simulink model "deadbeat_smm_with_lqr"  (R2015a)
settings: Solver=FixedStepDiscrete  SolverMode=SingleTasking  StartTime=0.0  StopTime=inf  FixedStep=sample_time  RelTol=1e-3
undefined symbols (not defined in the file or in its folder): A_kalman_fourbar_gear, A_kalman_transverse, A_kalman_vertical, A_lpf_accelerometer, A_lpf_fourbar_angles, A_lpf_imu, A_lpf_lateral_angle, B1_lpf_accelerometer, B1_lpf_fourbar_angles, B1_lpf_imu, B1_lpf_lateral_angle, B2_lpf_accelerometer, B2_lpf_fourbar_angles, B2_lpf_imu, B2_lpf_lateral_angle, B_dx_versus_x0, B_kalman_fourbar_gear, B_kalman_transverse, B_kalman_vertical, backwards_K_sag_of_t, backwards_P_sag_of_t, C_kalman_fourbar_gear, C_kalman_transverse, C_kalman_vertical, com_leg_motor, com_torso, contact_threshold, control_start_time, d_ankle_to_foot, d_vertical_com, desired_com_forward_velocity, desired_com_lateral_velocity, desired_initial_leg_roll_left, desired_initial_leg_roll_right, desired_stance_beta2, desired_standing_torso_pitch, desired_standing_torso_roll, desired_standing_z, desired_torso_pitch, desired_torso_roll, Discrete, enable_bouncing, fcut_contact, fdesignblkfcn, forward_dx_of_dxstar, forward_x_of_dxstar, g, gcbh, HIP_MTR_MAX_CONT_TORQUE, HIP_MTR_MAX_TORQUE, i_leg_motor, i_robot, i_torso, initial_dx_estimate, initial_dy_estimate, initial_dz_estimate, initial_leg_selection, initial_z_estimate, k_lateral_accel_for_torso_roll, k_lateral_swing_on_boom ... (+77)
libraries: simulink x21, ctrlSharedLib x7, dsparch4 x3
(part 4 of 5)

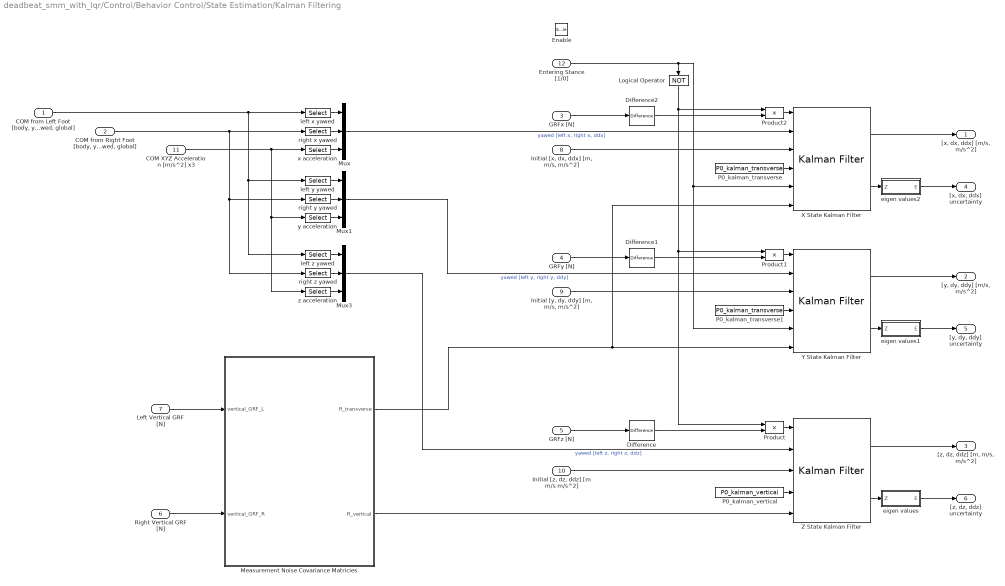
== system deadbeat_smm_with_lqr/Control/Behavior Control/State Estimation/Kalman Filtering ==
  "COM from Left Foot [body, yawed, global]" : Inport  SampleTime=sample_time
  "COM from Right Foot [body, yawed, global]" : Inport  Port=2  SampleTime=sample_time
  GRFx [N] : Inport  Port=3  SampleTime=sample_time
  GRFy [N] : Inport  Port=4  SampleTime=sample_time
  GRFz [N] : Inport  Port=5  SampleTime=sample_time
  Right Vertical GRF [N] : Inport  Port=6  SampleTime=sample_time
  Left Vertical GRF [N] : Inport  Port=7  SampleTime=sample_time
  "Initial [x, dx, ddx] [m, m/s, m/s^2]" : Inport  Port=8  PortDimensions=3  SampleTime=sample_time
  "Initial [y, dy, ddy] [m, m/s, m/s^2]" : Inport  Port=9  PortDimensions=3  SampleTime=sample_time
  "Initial [z, dz, ddz] [m m/s m/s^2]" : Inport  Port=10  PortDimensions=3  SampleTime=sample_time
  COM XYZ Acceleration [m/s^2] x3 : Inport  Port=11  SampleTime=sample_time
  Entering Stance [1/0] : Inport  Port=12  PortDimensions=1  SampleTime=sample_time
  Enable : EnablePort  StatesWhenEnabling=reset
  Difference : simulink/Discrete/Difference  ICPrevInput=0.0  InputProcessing=Inherited  OutMin=[]  OutMax=[]  OutDataType=fixdt(1, 16)  OutScaling=2^-10  DoSatur=off
  Difference1 : simulink/Discrete/Difference  ICPrevInput=0.0  InputProcessing=Inherited  OutMin=[]  OutMax=[]  OutDataType=fixdt(1, 16)  OutScaling=2^-10  DoSatur=off
  Difference2 : simulink/Discrete/Difference  ICPrevInput=0.0  InputProcessing=Inherited  OutMin=[]  OutMax=[]  OutDataType=fixdt(1, 16)  OutScaling=2^-10  DoSatur=off
  Logical Operator : Logic  Operator=NOT  AllPortsSameDT=off  OutDataTypeStr=boolean
  Measurement Noise Covariance Matricies : MATLAB Function  TreatAsAtomicUnit=on
  Mux : Mux  Inputs=3
  Mux1 : Mux  Inputs=3
  Mux3 : Mux  Inputs=3
  P0_kalman_transverse : Constant  Value=P0_kalman_transverse
  P0_kalman_transverse1 : Constant  Value=P0_kalman_transverse
  P0_kalman_vertical : Constant  Value=P0_kalman_vertical
  Product : Product
  Product1 : Product
  Product2 : Product
  X State Kalman Filter : ctrlSharedLib/Kalman Filter  TimeDomain=Discrete-Time  UseCurrentEstimator=on  ModelSource=Individual A, B, C, D matrices  ModelSourceVariable=A_kf  A=A_kalman_transverse  B=B_kalman_transverse  C=C_kalman_transverse  D=0  NumberOfStates=2  NumberOfInputs=1  NumberOfOutputs=2  InitialEstimateSource=Input port  X0=initial_dx_estimate  P0=P0_kalman_transverse  UseK=off  UseGH=on  NumberOfProcessNoiseInputs=1  G=G_kalman_transverse  TimeInvariantG=on  H=0  TimeInvariantH=on  Q=Q_kalman_GRF_difference  TimeInvariantQ=on  R=1  TimeInvariantR=off  N=0  TimeInvariantN=on  AddInputPort=on  AddEnablePort=off  ExternalReset=Rising  OutputEstimatedY=off  OutputP=on  Ts=sample_time
  Y State Kalman Filter : ctrlSharedLib/Kalman Filter  TimeDomain=Discrete-Time  UseCurrentEstimator=on  ModelSource=Individual A, B, C, D matrices  ModelSourceVariable=A_kf  A=A_kalman_transverse  B=B_kalman_transverse  C=C_kalman_transverse  D=0  NumberOfStates=2  NumberOfInputs=1  NumberOfOutputs=2  InitialEstimateSource=Input port  X0=initial_dy_estimate  P0=P0_kalman_transverse  UseK=off  UseGH=on  NumberOfProcessNoiseInputs=1  G=G_kalman_transverse  TimeInvariantG=on  H=0  TimeInvariantH=on  Q=Q_kalman_GRF_difference  TimeInvariantQ=on  R=1  TimeInvariantR=off  N=0  TimeInvariantN=on  AddInputPort=on  AddEnablePort=off  ExternalReset=Rising  OutputEstimatedY=off  OutputP=on  Ts=sample_time
  Z State Kalman Filter : ctrlSharedLib/Kalman Filter  TimeDomain=Discrete-Time  UseCurrentEstimator=on  ModelSource=Individual A, B, C, D matrices  ModelSourceVariable=A_kf  A=A_kalman_vertical  B=B_kalman_vertical  C=C_kalman_vertical  D=0  NumberOfStates=2  NumberOfInputs=1  NumberOfOutputs=2  InitialEstimateSource=Input port  X0=[initial_z_estimate; initial_dz_estimate]  P0=P0_kalman_vertical  UseK=off  UseGH=on  NumberOfProcessNoiseInputs=1  G=G_kalman_vertical  TimeInvariantG=on  H=0  TimeInvariantH=on  Q=Q_kalman_GRF_difference  TimeInvariantQ=on  R=1  TimeInvariantR=off  N=0  TimeInvariantN=on  AddInputPort=on  AddEnablePort=off  OutputEstimatedY=off  OutputP=on  Ts=sample_time
  eigen values : MATLAB Function  TreatAsAtomicUnit=on
  eigen values1 : MATLAB Function  TreatAsAtomicUnit=on
  eigen values2 : MATLAB Function  TreatAsAtomicUnit=on
  left x yawed : Selector  InputPortWidth=9  Indices=[4]
  left y yawed : Selector  InputPortWidth=9  Indices=[5]
  left z yawed : Selector  InputPortWidth=9  Indices=[6]
  right x yawed : Selector  InputPortWidth=9  Indices=[4]
  right y yawed : Selector  InputPortWidth=9  Indices=[5]
  right z yawed : Selector  InputPortWidth=9  Indices=[6]
  x acceleration : Selector  InputPortWidth=3  Indices=[1]
  y acceleration : Selector  InputPortWidth=3  Indices=[2]
  z acceleration : Selector  InputPortWidth=3  Indices=[3]
  "[x, dx, ddx] [m/s, m/s^2]" : Outport
  "[y, dy, ddy] [m/s, m/s^2]" : Outport  Port=2
  "[z, dz, ddz] [m, m/s, m/s^2]" : Outport  Port=3
  "[x, dx, ddx] uncertainty" : Outport  Port=4
  "[y, dy, ddy] uncertainty" : Outport  Port=5
  "[z, dz, ddz] uncertainty" : Outport  Port=6
  wires:
  X State Kalman Filter/1 -> "[x, dx, ddx] [m/s, m/s^2]"/1
  eigen values1/1(E) -> "[y, dy, ddy] uncertainty"/1
  eigen values2/1(E) -> "[x, dx, ddx] uncertainty"/1
  Y State Kalman Filter/1 -> "[y, dy, ddy] [m/s, m/s^2]"/1
  y acceleration/1 -> Mux1/3
  x acceleration/1 -> Mux/3
  z acceleration/1 -> Mux3/3
  COM XYZ Acceleration [m/s^2] x3/1 -> z acceleration/1, y acceleration/1, x acceleration/1
  Z State Kalman Filter/1 -> "[z, dz, ddz] [m, m/s, m/s^2]"/1
  GRFy [N]/1 -> Difference1/1
  Mux3/1 -> Z State Kalman Filter/2  "yawed [left z, right z, ddz]"
  GRFx [N]/1 -> Difference2/1
  Measurement Noise Covariance Matricies/2(R_vertical) -> Z State Kalman Filter/5
  Measurement Noise Covariance Matricies/1(R_transverse) -> X State Kalman Filter/6, Y State Kalman Filter/6
  Mux1/1 -> Y State Kalman Filter/2  "yawed [left y, right y, ddy]"
  Mux/1 -> X State Kalman Filter/2  "yawed [left x, right x, ddx]"
  Right Vertical GRF [N]/1 -> Measurement Noise Covariance Matricies/2(vertical_GRF_R)
  Left Vertical GRF [N]/1 -> Measurement Noise Covariance Matricies/1(vertical_GRF_L)
  "COM from Left Foot [body, yawed, global]"/1 -> left z yawed/1, left y yawed/1, left x yawed/1
  left x yawed/1 -> Mux/1
  "COM from Right Foot [body, yawed, global]"/1 -> right z yawed/1, right y yawed/1, right x yawed/1
  right x yawed/1 -> Mux/2
  left y yawed/1 -> Mux1/1
  right y yawed/1 -> Mux1/2
  left z yawed/1 -> Mux3/1
  right z yawed/1 -> Mux3/2
  P0_kalman_transverse/1 -> X State Kalman Filter/4
  "Initial [x, dx, ddx] [m, m/s, m/s^2]"/1 -> X State Kalman Filter/3
  P0_kalman_transverse1/1 -> Y State Kalman Filter/4
  "Initial [y, dy, ddy] [m, m/s, m/s^2]"/1 -> Y State Kalman Filter/3
  P0_kalman_vertical/1 -> Z State Kalman Filter/4
  "Initial [z, dz, ddz] [m m/s m/s^2]"/1 -> Z State Kalman Filter/3
  X State Kalman Filter/2 -> eigen values2/1(Z)
  Y State Kalman Filter/2 -> eigen values1/1(Z)
  Z State Kalman Filter/2 -> eigen values/1(Z)
  eigen values/1(E) -> "[z, dz, ddz] uncertainty"/1
  Logical Operator/1 -> Product2/1, Product/1, Product1/1
  Difference/1 -> Product/2
  Entering Stance [1/0]/1 -> Y State Kalman Filter/5, X State Kalman Filter/5, Logical Operator/1
  Difference1/1 -> Product1/2
  Difference2/1 -> Product2/2
  Product2/1 -> X State Kalman Filter/1
  Product1/1 -> Y State Kalman Filter/1
  Product/1 -> Z State Kalman Filter/1
  GRFz [N]/1 -> Difference/1

== system deadbeat_smm_with_lqr/Control/Behavior Control/State Estimation/Lowpass Filter ==
  In : Inport
  Generated Filter Block : dsparch4/Biquad Filter  Tag=BlockMethodSubSystem  IIRFiltStruct=Direct form II  CoeffSource=Specify via dialog  BiQuadCoeffs=[1.0218648663828083 -2 1.0218648663828083 1 -1.9114378222117407 0.91557643487411833]  a0Flag=Warning  IC=0  ICnum=0  ICden=0  denAccumFracLength=30  denProdOutputFracLength=30  secondMemoryFracLength=15  roundingMode=Floor  overflowMode=off  ScaleValues=[0.0041174265739107223;22.985401576126357]  optimizeScaleValues=off  ScaleValueMode=Specify via input port (g)  scaleValueFracLength=14  FilterSource=Specify via dialog  FilterObject=Hm_biquad
  Out : Outport
  wires:
  In/1 -> Generated Filter Block/1
  Generated Filter Block/1 -> Out/1

== system deadbeat_smm_with_lqr/Control/Behavior Control/Primary and Lateral Behavior/Circular Buffer/Enabled on Touchdown ==
  In : Inport
  Enable : EnablePort
  Out : Outport
  wires:
  In/1 -> Out/1

== system deadbeat_smm_with_lqr/Control/Behavior Control/Primary and Lateral Behavior/Flight/Back//Front PD ==
  Desired Position [rad] [back front] : Inport
  Desired Velocity [rad/s] [back front] : Inport  Port=2
  Measured Position [rad] [back front] : Inport  Port=3
  Measured Velocity [rad/s] [back front] : Inport  Port=4
  Back Tracking : Scope  NumInputPorts=2
      settings: YMin=3.725~-1  YMax=4.05~0.9  SaveName=ScopeData6  SampleInput=on
  Front Tracking : Scope  NumInputPorts=2
      settings: YMin=-1~-0.8  YMax=1~1.4  SaveName=ScopeData31  SampleInput=on
  Kp_SEA_Trajectory : Constant  Value=kp_velocity_swing_trajectory
  Mux{1..2,12..13} (4 alike) : Mux  Inputs=2
  Product1 : Product
  Selector{,1..3} (4 alike) : Selector  InputPortWidth=2  Indices=[1]
  Selector{4..7} (4 alike) : Selector  InputPortWidth=2  Indices=[2]
  Sum7 : Sum  Inputs=|+-
  Sum9 : Sum
  Commanded Velocity [rad/s] [back front] : Outport
  wires:
  Kp_SEA_Trajectory/1 -> Product1/2
  Sum9/1 -> Commanded Velocity [rad/s] [back front]/1
  Measured Velocity [rad/s] [back front]/1 -> Selector7/1, Selector3/1
  Desired Velocity [rad/s] [back front]/1 -> Selector6/1, Selector2/1, Sum9/2
  Measured Position [rad] [back front]/1 -> Selector4/1, Selector/1, Sum7/2
  Sum7/1 -> Product1/1
  Product1/1 -> Sum9/1
  Mux12/1 -> Back Tracking/2
  Mux13/1 -> Back Tracking/1
  Desired Position [rad] [back front]/1 -> Selector5/1, Selector1/1, Sum7/1
  Mux1/1 -> Front Tracking/2
  Mux2/1 -> Front Tracking/1
  Selector/1 -> Mux13/1
  Selector1/1 -> Mux13/2
  Selector2/1 -> Mux12/1
  Selector3/1 -> Mux12/2
  Selector5/1 -> Mux2/2
  Selector4/1 -> Mux2/1
  Selector6/1 -> Mux1/1
  Selector7/1 -> Mux1/2

== system deadbeat_smm_with_lqr/Control/Behavior Control/Primary and Lateral Behavior/Flight/Hold Values on Takeoff ==
  in : Inport
  Trigger : TriggerPort  ShowOutputPort=on  PortDimensions=1
  Subsystem : Subsystem
  out : Outport
  wires:
  in/1 -> Subsystem/1(in)
  Subsystem/1(out) -> out/1
  Trigger/1 -> Subsystem/Enable

== system deadbeat_smm_with_lqr/Control/Behavior Control/Primary and Lateral Behavior/Stance/Chirp Frequency ==
  Time Since Stance : Inport
  Chirp Freq Factor Saturation : Saturate  UpperLimit=standing_bounce_max_chirp_scale  LowerLimit=0
      settings: AttributesFormatString=Top: %<UpperLimit>\nBottom: %<LowerLimit>
  Compare To Constant1 : simulink/Logic and Bit Operations/Compare To Constant  relop=~=  const=standing_bounce_max_chirp_scale  OutDataTypeStr=boolean
  Constant1 : Constant
  Constant5 : Constant  Value=standing_bounce_increase_rate
  Product{1..4} (4 alike) : Product
  Sum : Sum  Inputs=++|
  standing_bounce_frequency : Constant  Value=standing_bounce_frequency
  w : Outport
  dw/dt : Outport  Port=2
  wires:
  standing_bounce_frequency/1 -> Product2/1, Product3/1
  Chirp Freq Factor Saturation/1 -> Product3/2, Compare To Constant1/1
  Product3/1 -> w/1
  Product1/1 -> dw/dt/1
  Compare To Constant1/1 -> Product1/1
  Product2/1 -> Product1/2
  Constant5/1 -> Product2/2, Product4/2
  Time Since Stance/1 -> Product4/1
  Sum/1 -> Chirp Freq Factor Saturation/1
  Product4/1 -> Sum/2
  Constant1/1 -> Sum/1

== system deadbeat_smm_with_lqr/Control/Behavior Control/Primary and Lateral Behavior/Stance/Compute Forces1 ==
  XYZ Acceleration : Inport
  Constant5 : Constant  Value=g
  Demux : Demux  Outputs=3
  Gain4 : Gain  Gain=m_total_real
  Mux : Mux  Inputs=3
  Sum8 : Sum  Inputs=|++
  XYZ Force : Outport
  wires:
  Constant5/1 -> Sum8/2
  XYZ Acceleration/1 -> Demux/1
  Gain4/1 -> XYZ Force/1
  Mux/1 -> Gain4/1
  Sum8/1 -> Mux/3
  Demux/3 -> Sum8/1
  Demux/2 -> Mux/2
  Demux/1 -> Mux/1

== system deadbeat_smm_with_lqr/Control/Behavior Control/Primary and Lateral Behavior/Stance/Hold Values on Takeoff ==
  in : Inport
  Trigger : TriggerPort  ShowOutputPort=on  PortDimensions=1
  Subsystem : Subsystem
  out : Outport
  wires:
  Trigger/1 -> Subsystem/Enable
  Subsystem/1(out) -> out/1
  in/1 -> Subsystem/1(in)

== system deadbeat_smm_with_lqr/Control/Behavior Control/Primary and Lateral Behavior/Stance/Hold Values on Touchdown ==
  in : Inport
  Trigger : TriggerPort  ShowOutputPort=on  PortDimensions=1
  Subsystem : Subsystem
  out : Outport
  wires:
  in/1 -> Subsystem/1(in)
  Subsystem/1(out) -> out/1
  Trigger/1 -> Subsystem/Enable

== system deadbeat_smm_with_lqr/Control/Behavior Control/Primary and Lateral Behavior/Stance/Lowpass Filter ==
  In : Inport
  Generated Filter Block : dsparch4/Biquad Filter  Tag=BlockMethodSubSystem  IIRFiltStruct=Direct form II  CoeffSource=Specify via dialog  BiQuadCoeffs=[1.2169083457291219 -2 1.2169083457291219 1 -1.7334293610249598 0.76768521888208641]  a0Flag=Warning  IC=0  ICnum=0  ICden=0  denAccumFracLength=30  denProdOutputFracLength=30  secondMemoryFracLength=15  roundingMode=Floor  overflowMode=off  ScaleValues=[0.034049223021428709;2.3191101889079508]  optimizeScaleValues=off  ScaleValueMode=Specify via input port (g)  scaleValueFracLength=14  FilterSource=Specify via dialog  FilterObject=Hm_biquad
  Out : Outport
  wires:
  In/1 -> Generated Filter Block/1
  Generated Filter Block/1 -> Out/1

== system deadbeat_smm_with_lqr/Control/Behavior Control/Primary and Lateral Behavior/Stance/Torque Distribution ==
  Leg Torque [Nm] : Inport
  Leg Force [N] : Inport  Port=2
  w [m] : Inport  Port=3
  Gain : Gain  Gain=0.5
  Gain1 : Gain  Gain=0.5
  Motor Torque Saturation Optimization : MATLAB Function  TreatAsAtomicUnit=on
  Product : Product  RndMeth=Zero
  Sum : Sum  Inputs=|++
  Sum1 : Sum  Inputs=+-|
  Back Torque [Nm] : Outport
  Front Torque [Nm] : Outport  Port=2
  wires:
  Gain/1 -> Motor Torque Saturation Optimization/1(x1s)
  Gain1/1 -> Motor Torque Saturation Optimization/2(x2s)
  Product/1 -> Gain1/1
  Leg Force [N]/1 -> Product/1
  Motor Torque Saturation Optimization/2(t2) -> Sum/2, Sum1/2
  w [m]/1 -> Product/2
  Motor Torque Saturation Optimization/1(t1) -> Sum1/1, Sum/1
  Sum/1 -> Front Torque [Nm]/1
  Leg Torque [Nm]/1 -> Gain/1
  Sum1/1 -> Back Torque [Nm]/1

== system deadbeat_smm_with_lqr/Control/Behavior Control/Primary and Lateral Behavior/Flight/Hold Values on Takeoff/Subsystem ==
  in : Inport
  Enable : EnablePort
  out : Outport
  wires:
  in/1 -> out/1

== system deadbeat_smm_with_lqr/Control/Behavior Control/Primary and Lateral Behavior/Stance/Hold Values on Takeoff/Subsystem ==
  in : Inport
  Enable : EnablePort
  out : Outport
  wires:
  in/1 -> out/1

== system deadbeat_smm_with_lqr/Control/Behavior Control/Primary and Lateral Behavior/Stance/Hold Values on Touchdown/Subsystem ==
  in : Inport
  Enable : EnablePort
  out : Outport
  wires:
  in/1 -> out/1

== matlab function deadbeat_smm_with_lqr/Control/Behavior Control/Compute World Frame COM Coordinates from Yawed Frame ==
  data: com_position_world output; X_dX input; Y_dY input; Z_dZ input; torso_yaw input; com_velocity_world output
function [com_position_world, com_velocity_world] ...
          = compute_com_state_in_world_frame(X_dX, Y_dY, Z_dZ, torso_yaw)

    R_yawed_to_world = R_yaw(torso_yaw(1));
    dR_yawed_to_world = dR_yaw(torso_yaw(1),torso_yaw(2));
    
    com_position_yawed = [X_dX(1); Y_dY(1); Z_dZ(1)];
    com_velocity_yawed = [X_dX(2); Y_dY(2); Z_dZ(2)];
    
    com_position_world = R_yawed_to_world*com_position_yawed;
    com_velocity_world = dR_yawed_to_world*com_position_yawed + R_yawed_to_world*com_velocity_yawed;

end

function R_gy = R_yaw(psi) % map yawed frame to global
  R_gy = [cos(psi), -sin(psi), 0; sin(psi), cos(psi), 0; 0 0 1]; 
end
function dR_gy = dR_yaw(psi,dpsi)
  dR_gy = dpsi*[-sin(psi), -cos(psi), 0; cos(psi), -sin(psi), 0; 0 0 0];
end

== matlab function deadbeat_smm_with_lqr/Control/Behavior Control/Primary and Lateral Behavior/Stance/2D Lateral Stance Control ==
  data: F_leg input; lateral_torque output; lateral_offset parameter; m_total_real parameter; m_leg_motor parameter; m_leg parameter
function lateral_torque = lateralStanceControl2D(F_leg,lateral_offset,m_total_real,m_leg_motor,m_leg)
    lateral_torque = -F_leg*lateral_offset*(m_total_real-(m_leg_motor+m_leg))/m_total_real;
end

== matlab function deadbeat_smm_with_lqr/Control/Behavior Control/Atrias Swing control/Avoid Hitting Mechanical Limits ==
  data: back_cmd output double; front_cmd output double; dback_cmd output double; dfront_cmd output double; ddback_cmd output double; ddfront_cmd output double; back_desired input; dback_desired input; ddback_desired input; front_desired input; dfront_desired input; ddfront_desired input; min_front_bar_angle parameter; max_front_bar_angle parameter; min_back_bar_angle parameter; max_back_bar_angle parameter
%% Avoid joint limits by ensuring we don't command velocities/accelerations that would push us into them when we are close to them.
function [back_cmd, front_cmd, dback_cmd, dfront_cmd, ddback_cmd, ddfront_cmd] ...
    = AvoidFourbarLimits(back_desired,dback_desired, ddback_desired, ...
          front_desired, dfront_desired, ddfront_desired, ...
          min_front_bar_angle, max_front_bar_angle, min_back_bar_angle, max_back_bar_angle)
    [back_cmd, front_cmd, dback_cmd, dfront_cmd, ddback_cmd, ddfront_cmd] = AvoidFourbarLimits(back_desired,dback_desired, ddback_desired, front_desired, dfront_desired, ddfront_desired, min_front_bar_angle, max_front_bar_angle, min_back_bar_angle, max_back_bar_angle);
end

== matlab function deadbeat_smm_with_lqr/Control/Behavior Control/Atrias Swing control/Convert COM Position to Joint Angles + Leg Length  ==
  data: desired_leg_length output; X_star input; Y_star input; Z_star input; right_left input; com_pelvis_body input; desired_alpha output; desired_beta output; dcom_pelvis_body input; roll input; pitch input; sagittal_angle input; lateral_angle input; leg_length input; lateral_offset parameter; minimum_lateral_beta parameter; maximum_lateral_beta parameter
function [ desired_leg_length, desired_alpha, desired_beta ]  =  ...
          ConvertToJointAnglesAndLegLength(X_star, Y_star, Z_star, right_left,...
                           com_pelvis_body, dcom_pelvis_body, ...
                           roll, pitch, sagittal_angle, lateral_angle, leg_length,...
                           lateral_offset, minimum_lateral_beta, maximum_lateral_beta) 

    q = [roll(1), pitch(1), sagittal_angle(1), lateral_angle(1), leg_length(1)];
    dq = [roll(2), pitch(2), sagittal_angle(2), lateral_angle(2), leg_length(2)];
    [desired_alpha, desired_beta, desired_leg_length]  =  ConvertComPositionToLegAnglesAndLegLength(X_star, Y_star, Z_star, right_left, com_pelvis_body, dcom_pelvis_body, q, dq, lateral_offset);   
    desired_beta = saturate(desired_beta, minimum_lateral_beta, maximum_lateral_beta);
end

function [desired_saturated] = saturate(desired, minimum_lateral_beta, maximum_lateral_beta)
    desired_saturated = desired;
    if desired(1) < minimum_lateral_beta
        desired_saturated = [minimum_lateral_beta; 0; 0];
    elseif desired(1) > maximum_lateral_beta
        desired_saturated = [maximum_lateral_beta; 0; 0];    
    end
end

== matlab function deadbeat_smm_with_lqr/Control/Behavior Control/Atrias Swing control/Virtual Leg to Four Bar ==
  data: l_leg input; dl_leg input; ddl_leg input; phi input; dphi input; ddphi input; back output; dback output; ddback output; front output; dfront output; ddfront output
function [back, dback, ddback, front, dfront, ddfront] = VirtualLegToFourBar(l_leg, dl_leg, ddl_leg, phi, dphi, ddphi)
    [back, dback, ddback, front, dfront, ddfront] = VirtualLegToFourBar(l_leg, dl_leg, ddl_leg, phi, dphi, ddphi);
end

== stateflow chart deadbeat_smm_with_lqr/Control/Behavior Control/Contact State Machine/State Machine ==
  state TouchDown
  state LockedContact
  state Unloading
  state Takeoff
  state Flight
  (junction 91) -> TouchDown
  TouchDown -> (junction 130) [order 2] : [vertical_grf < contact_threshold]
  (junction 93) -> (junction 91)
  (junction 130) -> (junction 128)
  TouchDown -> LockedContact [order 1] : [vertical_grf > loaded_threshold]
  (junction 115) -> LockedContact
  (junction 118) -> (junction 115)
  LockedContact -> Unloading : [z_velocity >= 0 && previous_z_velocity < 0]
  Unloading -> LockedContact [order 2] : [vertical_grf > loaded_threshold && z_velocity < 0]
  (junction 122) -> (junction 118)
  Unloading -> Takeoff [order 1] : [vertical_grf < contact_threshold]
  Takeoff -> Flight : after(t_flight,sec)
  (default) -> Flight
  Flight -> (junction 93) : [vertical_grf > contact_threshold]
  (junction 128) -> Flight
  data: z_velocity input; previous_z_velocity input; vertical_grf input; t_flight parameter; g parameter; contact_threshold parameter; loaded_threshold parameter; TouchDown output boolean; LockedContact output boolean; Unloading output boolean; Takeoff output boolean; Flight output boolean; vertical_acceleration input

== matlab function deadbeat_smm_with_lqr/Control/Behavior Control/Force Estimation/3D Forward Dynamics yawed ==
  data: right_or_left input; torso_roll input size=2; torso_pitch input double size=2; torso_yaw input double size=2; primary_sagittal_leg_angle input double size=2; primary_leg_length input double size=2; primary_leg_roll input double size=2; secondary_leg_roll input double size=2; primary_leg_torque input; primary_leg_force input; primary_lateral_torque input; secondary_lateral_torque input; R_GRF output double size=3; L_GRF output size=3; ddroll output double; g parameter; m_leg_motor parameter; m_torso parameter; i_torso parameter; i_leg_motor parameter; lateral_offset parameter; com_torso parameter; torso_centerline_roll_offset_angle parameter
%% Forward 3D ATRIAS dynamics
function [R_GRF, L_GRF, ddroll]  =  ForwardDynamics3D(right_or_left, ...
                                                      torso_roll, torso_pitch, torso_yaw, ...
                                                      primary_sagittal_leg_angle, primary_leg_length,...
                                                      primary_leg_roll, secondary_leg_roll, ...
                                                      primary_leg_torque, primary_leg_force, ...
                                                      primary_lateral_torque, secondary_lateral_torque, ...
                                                      g, m_leg_motor, m_torso, i_torso, i_leg_motor, lateral_offset, com_torso, torso_centerline_roll_offset_angle)

    d = norm(com_torso(2:3));
    It = mean(i_torso);
    Im = mean(i_leg_motor);
    
    phi    = torso_roll(1) + torso_centerline_roll_offset_angle;  % roll
    theta  = torso_pitch(1);                   % pitch
    alpha1 = primary_sagittal_leg_angle(1);    % primary sagittal leg angle
    beta1  = primary_leg_roll(1);              % primary leg roll
    beta2  = secondary_leg_roll(1);            % secondary leg roll
    if right_or_left
        beta1 = beta1 - torso_centerline_roll_offset_angle;
        beta2 = beta2 + torso_centerline_roll_offset_angle;
    else
        beta1 = beta1 + torso_centerline_roll_offset_angle;
        beta2 = beta2 - torso_centerline_roll_offset_angle;
    end 
    l1     = primary_leg_length(1);            % primary leg length
    
    dphi    = torso_roll(2);
    dtheta  = torso_pitch(2);
    dpsi    = torso_yaw(2);
    dalpha1 = primary_sagittal_leg_angle(2);
    dbeta1  = primary_leg_roll(2);
    dbeta2  = secondary_leg_roll(2);
    dl1     = primary_leg_length(2);
    
    
    tau_a1 = primary_leg_torque;
    tau_b1 = primary_lateral_torque;
    tau_b2 = secondary_lateral_torque;
    F_l1 = primary_leg_force;

    if right_or_left == 1
      A = A_fwd_yawed_right(lateral_offset,d,m_leg_motor,m_torso,It,Im,phi,theta,alpha1,beta1,beta2,l1);
      B = B_fwd_yawed_right(lateral_offset,d,g,m_leg_motor,m_torso,It,Im,phi,theta,alpha1,beta1,beta2,l1,dphi,dtheta,dpsi,dalpha1,dbeta1,dbeta2,dl1,tau_a1,tau_b1,tau_b2,F_l1);
    else
      A = A_fwd_yawed_left(lateral_offset,d,m_leg_motor,m_torso,It,Im,phi,theta,alpha1,beta1,beta2,l1);
      B = B_fwd_yawed_left(lateral_offset,d,g,m_leg_motor,m_torso,It,Im,phi,theta,alpha1,beta1,beta2,l1,dphi,dtheta,dpsi,dalpha1,dbeta1,dbeta2,dl1,tau_a1,tau_b1,tau_b2,F_l1);
    end
    
    x_fwd = A \ B;
    ddroll = x_fwd(4);
    GRF = zeros(3,1);
    GRF(1) = x_fwd(11);
    GRF(2) = x_fwd(12);
    GRF(3) = x_fwd(13); 
    
    if right_or_left == 1
        R_GRF = GRF;
        L_GRF = [0;0;0];
    else
        R_GRF = [0;0;0];
        L_GRF = GRF;
    end
end

== matlab function deadbeat_smm_with_lqr/Control/Behavior Control/Force Estimation/Leg Force Measurements/Nonlinear Spring Force ==
  data: deflections input; tau_sea output
function tau_sea   = SeaSpringForce( deflections )
    tau_sea = SeaSpringForce( deflections );
end

== matlab function deadbeat_smm_with_lqr/Control/Behavior Control/Knee Torques ==
  data: right_knees_to_foot input; right_front_knee_torques_from_fd output; left_knees_to_foot input; grf_from_seas input; grf_from_accelerometer input; right_back_knee_torques_from_fd output; right_front_knee_torques_from_accelerometer output; right_back_knee_torques_from_accelerometer output; left_front_knee_torques_from_fd output; left_back_knee_torques_from_fd output; left_front_knee_torques_from_accelerometer output; left_back_knee_torques_from_accelerometer output
function [right_front_knee_torques_from_fd, right_back_knee_torques_from_fd,...
          right_front_knee_torques_from_accelerometer, right_back_knee_torques_from_accelerometer,...
          left_front_knee_torques_from_fd, left_back_knee_torques_from_fd,...
          left_front_knee_torques_from_accelerometer, left_back_knee_torques_from_accelerometer] ...
          = compute_knee_torques(right_knees_to_foot, left_knees_to_foot, grf_from_seas, grf_from_accelerometer)

      right_front_knee_torques_from_fd = cross(right_knees_to_foot(1:3), grf_from_seas);
      right_back_knee_torques_from_fd = cross(right_knees_to_foot(4:6), grf_from_seas);
      right_front_knee_torques_from_accelerometer = cross(right_knees_to_foot(1:3), grf_from_accelerometer);
      right_back_knee_torques_from_accelerometer = cross(right_knees_to_foot(4:6), grf_from_accelerometer);
      
      left_front_knee_torques_from_fd = cross(left_knees_to_foot(1:3), grf_from_seas);
      left_back_knee_torques_from_fd = cross(left_knees_to_foot(4:6), grf_from_seas);
      left_front_knee_torques_from_accelerometer = cross(left_knees_to_foot(1:3), grf_from_accelerometer);
      left_back_knee_torques_from_accelerometer = cross(left_knees_to_foot(4:6), grf_from_accelerometer);
end

== matlab function deadbeat_smm_with_lqr/Control/Behavior Control/Primary Secondary Leg Swap/ToggleRightLeftLeg ==
  data: toggle input boolean; right_left output double; previous_right_left input double
function right_left = ToggleRightLeftLeg(toggle, previous_right_left)
    
    if toggle
        right_left = -previous_right_left + 1;
    else
        right_left = previous_right_left;
    end

end

== matlab function deadbeat_smm_with_lqr/Control/Behavior Control/Primary and Lateral Behavior/Circular Buffer/Buffer ==
  data: data input; buffer output size=recorded_steps; trigger input; buffer_size input
function buffer  = buffer_data(data, trigger, buffer_size)

    persistent buffer_memory
    coder.varsize('buffer_memory',100);
    if isempty(buffer_memory)
        buffer_memory = [];
    end
    
    if trigger
        buffer_memory = [data; buffer_memory];
        if size(buffer_memory, 1) > buffer_size
            buffer_memory = buffer_memory(1:buffer_size,:);
        end
    end
    
    buffer = buffer_memory;

end

== matlab function deadbeat_smm_with_lqr/Control/Behavior Control/Primary and Lateral Behavior/Circular Buffer/Buffer1 ==
  data: data input; buffer output size=recorded_steps; trigger input; buffer_size input
function buffer  = buffer_data(data, trigger, buffer_size)

    persistent buffer_memory
    coder.varsize('buffer_memory',100);
    if isempty(buffer_memory)
        buffer_memory = [];
    end
    
    if trigger
        buffer_memory = [data; buffer_memory];
        if size(buffer_memory, 1) > buffer_size
            buffer_memory = buffer_memory(1:buffer_size,:);
        end
    end
    
    buffer = buffer_memory;

end

== matlab function deadbeat_smm_with_lqr/Control/Behavior Control/Primary and Lateral Behavior/Circular Buffer/Buffer2 ==
  data: data input; buffer output size=recorded_steps; trigger input; buffer_size input
function buffer  = buffer_data(data, trigger, buffer_size)

    persistent buffer_memory
    coder.varsize('buffer_memory',100);
    if isempty(buffer_memory)
        buffer_memory = [];
    end
    
    if trigger
        buffer_memory = [data; buffer_memory];
        if size(buffer_memory, 1) > buffer_size
            buffer_memory = buffer_memory(1:buffer_size,:);
        end
    end
    
    buffer = buffer_memory;

end

== matlab function deadbeat_smm_with_lqr/Control/Behavior Control/Primary and Lateral Behavior/Circular Buffer/Buffer3 ==
  data: data input; buffer output size=recorded_steps; trigger input; buffer_size input
function buffer  = buffer_data(data, trigger, buffer_size)

    persistent buffer_memory
    coder.varsize('buffer_memory',100);
    if isempty(buffer_memory)
        buffer_memory = [];
    end
    
    if trigger
        buffer_memory = [data; buffer_memory];
        if size(buffer_memory, 1) > buffer_size
            buffer_memory = buffer_memory(1:buffer_size,:);
        end
    end
    
    buffer = buffer_memory;

end

== matlab function deadbeat_smm_with_lqr/Control/Behavior Control/Primary and Lateral Behavior/Circular Buffer/Buffer4 ==
  data: data input; buffer output size=recorded_steps; trigger input; buffer_size input
function buffer  = buffer_data(data, trigger, buffer_size)

    persistent buffer_memory
    coder.varsize('buffer_memory',100);
    if isempty(buffer_memory)
        buffer_memory = [];
    end
    
    if trigger
        buffer_memory = [data; buffer_memory];
        if size(buffer_memory, 1) > buffer_size
            buffer_memory = buffer_memory(1:buffer_size,:);
        end
    end
    
    buffer = buffer_memory;

end

== matlab function deadbeat_smm_with_lqr/Control/Behavior Control/Primary and Lateral Behavior/Circular Buffer/Buffer5 ==
  data: data input; buffer output size=recorded_steps; trigger input; buffer_size input
function buffer  = buffer_data(data, trigger, buffer_size)

    persistent buffer_memory
    coder.varsize('buffer_memory',100);
    if isempty(buffer_memory)
        buffer_memory = [];
    end
    
    if trigger
        buffer_memory = [data; buffer_memory];
        if size(buffer_memory, 1) > buffer_size
            buffer_memory = buffer_memory(1:buffer_size,:);
        end
    end
    
    buffer = buffer_memory;

end

== matlab function deadbeat_smm_with_lqr/Control/Behavior Control/Primary and Lateral Behavior/Circular Buffer/Buffer6 ==
  data: data input; buffer output size=recorded_steps; trigger input; buffer_size input
function buffer  = buffer_data(data, trigger, buffer_size)

    persistent buffer_memory
    coder.varsize('buffer_memory',100);
    if isempty(buffer_memory)
        buffer_memory = [];
    end
    
    if trigger
        buffer_memory = [data; buffer_memory];
        if size(buffer_memory, 1) > buffer_size
            buffer_memory = buffer_memory(1:buffer_size,:);
        end
    end
    
    buffer = buffer_memory;

end

== matlab function deadbeat_smm_with_lqr/Control/Behavior Control/Primary and Lateral Behavior/Circular Buffer/Buffer7 ==
  data: data input; buffer output size=recorded_steps; trigger input; buffer_size input
function buffer  = buffer_data(data, trigger, buffer_size)

    persistent buffer_memory
    coder.varsize('buffer_memory',100);
    if isempty(buffer_memory)
        buffer_memory = [];
    end
    
    if trigger
        buffer_memory = [data; buffer_memory];
        if size(buffer_memory, 1) > buffer_size
            buffer_memory = buffer_memory(1:buffer_size,:);
        end
    end
    
    buffer = buffer_memory;

end

== matlab function deadbeat_smm_with_lqr/Control/Behavior Control/Primary and Lateral Behavior/Closed Loop Compensation/CLOSED LOOP COMPENSATION X FOR VAIRABLE SPEED ==
  data: A_cl input; epsilon input; c input; delta_s_i input; dx_star input; B_cl input; delta_ux output
function delta_ux  = closed_loop_compensation_dxstar...
         (A_cl,epsilon, c, delta_s_i, dx_star, B_cl)
% assume form of delta_s_{i+1} = A_cl*delta_s_i + epsilon +c*dx_star + B_cl*delta_ux
% where delta measures deviation from deadbeat case. solve for
% delta_ux = (-A_cl*delta_s_i-epsilon - c*dxstar)/B_cl to achieve deadbeat
delta_ux = (-A_cl*delta_s_i - epsilon - c*dx_star)/B_cl;

== matlab function deadbeat_smm_with_lqr/Control/Behavior Control/Primary and Lateral Behavior/Closed Loop Compensation/CLOSED LOOP COMPENSATION Y FOR VAIRABLE SPEED ==
  data: A_cl input; epsilon input; c input; delta_s_i input; dx_star input; B_cl input; delta_ux output
function delta_ux  = closed_loop_compensation_dxstar...
         (A_cl,epsilon, c, delta_s_i, dx_star, B_cl)
% assume form of delta_s_{i+1} = A_cl*delta_s_i + epsilon +c*dx_star + B_cl*delta_ux
% where delta measures deviation from deadbeat case. solve for
% delta_ux = (-A_cl*delta_s_i-epsilon - c*dxstar)/B_cl to achieve deadbeat
delta_ux = (-A_cl*delta_s_i - epsilon - c*dx_star)/B_cl;

== matlab function deadbeat_smm_with_lqr/Fourbar Gearside Kalman Filter/SeaTorques1 ==
  data: deflections input; tau output; k_sea_high parameter
function tau = SeaSpringForce(deflections, k_sea_high)
    tau = SeaSpringForce(deflections, k_sea_high);
end

== matlab function deadbeat_smm_with_lqr/Fourbar Gearside Kalman Filter/External Trunk Torque Estimate ==
  data: grf_xz input; rotor_torque input; spring_torque input; tau_trunk output; torso_pitch input; d_vertical_com parameter; LEG_MTR_GEAR_RATIO parameter
function tau_trunk = tau_trunk(grf_xz, rotor_torque, spring_torque, torso_pitch, d_vertical_com, LEG_MTR_GEAR_RATIO )
    d = d_vertical_com;
    theta = torso_pitch;
    N = LEG_MTR_GEAR_RATIO;
    tau_trunk = sum(-rotor_torque + -(N-1)/N*spring_torque) + (-d*cos(theta)*grf_xz(1) + d*sin(theta)*grf_xz(2));
end

== matlab function deadbeat_smm_with_lqr/Fourbar Gearside Kalman Filter/Covariance Estimates ==
  data: spring_torque input; absolute_gear input; current_position_estimate input; state_uncertainty input; Q1 output; R1 output; Q2 output; R2 output; R_kalman_absolute_normal parameter; R_kalman_absolute_fail parameter; R_kalman_incremental_unloaded parameter; R_kalman_incremental_loaded parameter; kalman_load_to_deflect_transmission parameter; Q3 output; R3 output; Q4 output; R4 output; max_absolute_measurement_innovation parameter; k_sea_low parameter; Q_kalman_spring_torque parameter; Q_kalman_rotor_torque parameter; Q_kalman_trunk_torque parameter; sample_time parameter
function [Q1, R1, Q2, R2, Q3, R3, Q4, R4] = covariance( spring_torque, absolute_gear, current_position_estimate, state_uncertainty, R_kalman_absolute_normal, R_kalman_absolute_fail, R_kalman_incremental_unloaded, R_kalman_incremental_loaded, kalman_load_to_deflect_transmission, max_absolute_measurement_innovation, k_sea_low, Q_kalman_spring_torque, Q_kalman_rotor_torque, Q_kalman_trunk_torque, sample_time)

    persistent previous_absolute_gear
    if isempty(previous_absolute_gear)
        previous_absolute_gear = absolute_gear;
    end
    
    % Measurement covariance
    R_absolute = ones(4,1)*R_kalman_absolute_normal;
    dropped_out = previous_absolute_gear == absolute_gear;
    out_of_range = abs(current_position_estimate - absolute_gear) > max_absolute_measurement_innovation;
    R_absolute(dropped_out | out_of_range) = R_kalman_absolute_fail;
    
    R_incremental_scale = min(abs(spring_torque)/kalman_load_to_deflect_transmission, 1);
    R_incremental = R_incremental_scale*R_kalman_incremental_loaded + (1-R_incremental_scale)*R_kalman_incremental_unloaded;
    
    R1 = diag([R_absolute(1), R_incremental(1)])/sample_time;
    R2 = diag([R_absolute(2), R_incremental(2)])/sample_time;
    R3 = diag([R_absolute(3), R_incremental(3)])/sample_time;
    R4 = diag([R_absolute(4), R_incremental(4)])/sample_time;
    
    % Process noise covariance
    Q_spring_torque = k_sea_low.^2.*(state_uncertainty + R_kalman_absolute_normal) + Q_kalman_spring_torque;

    Q1 = diag([Q_spring_torque(1), Q_kalman_rotor_torque, Q_kalman_trunk_torque]);
    Q2 = diag([Q_spring_torque(2), Q_kalman_rotor_torque, Q_kalman_trunk_torque]);
    Q3 = diag([Q_spring_torque(3), Q_kalman_rotor_torque, Q_kalman_trunk_torque]);
    Q4 = diag([Q_spring_torque(4), Q_kalman_rotor_torque, Q_kalman_trunk_torque]);

    previous_absolute_gear = absolute_gear;
end

== matlab function deadbeat_smm_with_lqr/Fourbar Gearside Kalman Filter/eigen values 1 ==
  data: Z input; E output
function E = eigen(Z)
    E = real(eig(Z));
    E = sort(E);
end

== matlab function deadbeat_smm_with_lqr/Fourbar Gearside Kalman Filter/eigen values 2 ==
  data: Z input; E output
function E = eigen(Z)
    E = real(eig(Z));
    E = sort(E);
end

== matlab function deadbeat_smm_with_lqr/Fourbar Gearside Kalman Filter/eigen values 3 ==
  data: Z input; E output
function E = eigen(Z)
    E = real(eig(Z));
    E = sort(E);
end

== matlab function deadbeat_smm_with_lqr/Fourbar Gearside Kalman Filter/eigen values4  ==
  data: Z input; E output
function E = eigen(Z)
    E = real(eig(Z));
    E = sort(E);
end

== matlab function deadbeat_smm_with_lqr/Control/Behavior Control/Primary and Lateral Behavior/Closed Loop Compensation/ESTIMATE CLOSED LOOP ERROR X FOR VARIABLE SPEED ==
  data: dx_land_hist input; A_cl output; delta_ux_hist input; dx_lift_hist input; dx_star_hist input; B_dx_versus_x0 parameter; W_real input; epsilon_0 output; c output; A_cl_nb output; epsilon_0_nb output; c_nb output
function [A_cl, epsilon_0, c, ...
          A_cl_nb, epsilon_0_nb, c_nb] = error_fitting_dxstar...
         (dx_land_hist, delta_ux_hist, dx_lift_hist, dx_star_hist,...
          B_dx_versus_x0, W_real)
% data_length = min([length(dx_lift_hist), filter_length]);
data_length = length(dx_lift_hist);
assert(data_length < 100);
% add fake data
fake_dx_land_err_magnitude = 0.1; fake_dx_star_magnitude = 0.1;
[fgrid_dx_land_err, fgrid_dx_star, fgrid_dx_lift_err] = ...
    meshgrid(fake_dx_land_err_magnitude*[-1 1],fake_dx_star_magnitude*[-1 1],0);
fake_data_length = numel(fgrid_dx_land_err);
fake_dx_land_err = fgrid_dx_land_err(:);
fake_dx_star = fgrid_dx_star(:);
fake_dx_lift_err = fgrid_dx_lift_err(:);
fake_delta_ux = zeros(fake_data_length,1);
% assert(fake_data_length<100);
% assert(filter_length<100);
% fake_dx_land_err = linspace(-0.1, 0.1, fake_data_length)';
% fake_dx_lift_err = zeros(fake_data_length,1);
% fake_delta_ux = zeros(fake_data_length,1);
% fake_dx_star = linspace(-0.25, 0.25, fake_data_length)';
dx_land_err = [reshape(dx_land_hist(1:data_length)-dx_star_hist(1:data_length),...
                       data_length, 1); fake_dx_land_err];
dx_lift_err = [reshape(dx_lift_hist(1:data_length)-dx_star_hist(1:data_length),...
                       data_length, 1); fake_dx_lift_err];
dx_star = [reshape(dx_star_hist(1:data_length), data_length,1); fake_dx_star];
delta_ux = [reshape(delta_ux_hist(1:data_length), data_length, 1); fake_delta_ux];
% weighted least squares
W = diag([W_real*ones(1,data_length), ones(1,fake_data_length)]);
Y = dx_lift_err - B_dx_versus_x0*delta_ux;
X = [dx_land_err, dx_star, ones(data_length+fake_data_length,1)];
% linear regression for s_{i+1}-s0 = A_cl*(s_i-s0) + epsilon_0 + c(s0) + B*delta_u
% solve for Y = X*beta, beta column vector
beta_hat = (X'*W*X)\X'*W*Y;
W_nobias = diag([W_real*ones(1,data_length), 0.001*ones(1,fake_data_length)]);
beta_hat_nobias = (X'*W_nobias*X)\X'*W_nobias*Y;
A_cl = beta_hat(1);
c = beta_hat(2);
epsilon_0 = beta_hat(3);
A_cl_nb = beta_hat_nobias(1);
c_nb = beta_hat_nobias(2);
epsilon_0_nb = beta_hat_nobias(3);

== matlab function deadbeat_smm_with_lqr/Control/Behavior Control/Primary and Lateral Behavior/Closed Loop Compensation/ESTIMATE CLOSED LOOP ERROR Y FOR VARIABLE SPEED ==
  data: dx_land_hist input; A_cl output; delta_ux_hist input; dx_lift_hist input; dx_star_hist input; B_dx_versus_x0 parameter; W_real input; epsilon_0 output; c output; A_cl_nb output; epsilon_0_nb output; c_nb output
function [A_cl, epsilon_0, c, ...
          A_cl_nb, epsilon_0_nb, c_nb] = error_fitting_dxstar...
         (dx_land_hist, delta_ux_hist, dx_lift_hist, dx_star_hist,...
          B_dx_versus_x0, W_real)
% data_length = min([length(dx_lift_hist), filter_length]);
data_length = length(dx_lift_hist);
assert(data_length < 100);
% add fake data
fake_dx_land_err_magnitude = 0.1; fake_dx_star_magnitude = 0.1;
[fgrid_dx_land_err, fgrid_dx_star, fgrid_dx_lift_err] = ...
    meshgrid(fake_dx_land_err_magnitude*[-1 1],fake_dx_star_magnitude*[-1 1],0);
fake_data_length = numel(fgrid_dx_land_err);
fake_dx_land_err = fgrid_dx_land_err(:);
fake_dx_star = fgrid_dx_star(:);
fake_dx_lift_err = fgrid_dx_lift_err(:);
fake_delta_ux = zeros(fake_data_length,1);
% assert(fake_data_length<100);
% assert(filter_length<100);
% fake_dx_land_err = linspace(-0.1, 0.1, fake_data_length)';
% fake_dx_lift_err = zeros(fake_data_length,1);
% fake_delta_ux = zeros(fake_data_length,1);
% fake_dx_star = linspace(-0.25, 0.25, fake_data_length)';
dx_land_err = [reshape(dx_land_hist(1:data_length)-dx_star_hist(1:data_length),...
                       data_length, 1); fake_dx_land_err];
dx_lift_err = [reshape(dx_lift_hist(1:data_length)-dx_star_hist(1:data_length),...
                       data_length, 1); fake_dx_lift_err];
dx_star = [reshape(dx_star_hist(1:data_length), data_length,1); fake_dx_star];
delta_ux = [reshape(delta_ux_hist(1:data_length), data_length, 1); fake_delta_ux];
% weighted least squares
W = diag([W_real*ones(1,data_length), ones(1,fake_data_length)]);
Y = dx_lift_err - B_dx_versus_x0*delta_ux;
X = [dx_land_err, dx_star, ones(data_length+fake_data_length,1)];
% linear regression for s_{i+1}-s0 = A_cl*(s_i-s0) + epsilon_0 + c(s0) + B*delta_u
% solve for Y = X*beta, beta column vector
beta_hat = (X'*W*X)\X'*W*Y;
W_nobias = diag([W_real*ones(1,data_length), 0.001*ones(1,fake_data_length)]);
beta_hat_nobias = (X'*W_nobias*X)\X'*W_nobias*Y;
A_cl = beta_hat(1);
c = beta_hat(2);
epsilon_0 = beta_hat(3);
A_cl_nb = beta_hat_nobias(1);
c_nb = beta_hat_nobias(2);
epsilon_0_nb = beta_hat_nobias(3);

== matlab function deadbeat_smm_with_lqr/Control/Behavior Control/Primary and Lateral Behavior/Desired Forward Velocity ==
  data: dx_takeoff input; desired_dx output; desired_forward_velocity input; forward_velocity_target_step parameter
function desired_dx = dx_command(dx_takeoff, desired_forward_velocity, forward_velocity_target_step)
    desired_direction = sign(desired_forward_velocity);
    desired_dx = dx_takeoff + desired_direction*forward_velocity_target_step;
    desired_dx = max(min(desired_dx, abs(desired_forward_velocity)),-abs(desired_forward_velocity));
end

== matlab function deadbeat_smm_with_lqr/Control/Behavior Control/Primary and Lateral Behavior/Flight/Avoid Hitting Mechanical Limits ==
  data: back_cmd output double; front_cmd output double; dback_cmd output double; dfront_cmd output double; ddback_cmd output double; ddfront_cmd output double; back_desired input; dback_desired input; ddback_desired input; front_desired input; dfront_desired input; ddfront_desired input; min_front_bar_angle parameter; max_front_bar_angle parameter; min_back_bar_angle parameter; max_back_bar_angle parameter
%% Avoid joint limits by ensuring we don't command velocities/accelerations that would push us into them when we are close to them.
function [back_cmd, front_cmd, dback_cmd, dfront_cmd, ddback_cmd, ddfront_cmd] ...
    = AvoidFourbarLimits(back_desired,dback_desired, ddback_desired, ...
          front_desired, dfront_desired, ddfront_desired, ...
          min_front_bar_angle, max_front_bar_angle, min_back_bar_angle, max_back_bar_angle)
    [back_cmd, front_cmd, dback_cmd, dfront_cmd, ddback_cmd, ddfront_cmd] = AvoidFourbarLimits(back_desired,dback_desired, ddback_desired, front_desired, dfront_desired, ddfront_desired, min_front_bar_angle, max_front_bar_angle, min_back_bar_angle, max_back_bar_angle);
end

== matlab function deadbeat_smm_with_lqr/Control/Behavior Control/Primary and Lateral Behavior/Flight/Avoid Virtual Leg Length Limits ==
  data: l_leg_desired input; dl_leg_desired input; ddl_leg_desired input; l_leg_cmd output double; dl_leg_cmd output double; ddl_leg_cmd output double; min_leg_length parameter; max_leg_length parameter
%% Avoid virtual leg length limits by ensuring we don't command position/velocities/accelerations that would hit them.
function [l_leg_cmd, dl_leg_cmd, ddl_leg_cmd] = AvoidVirtualLengthLimits(l_leg_desired, dl_leg_desired, ddl_leg_desired, min_leg_length, max_leg_length)
    [l_leg_cmd, dl_leg_cmd, ddl_leg_cmd] = AvoidVirtualLengthLimits(l_leg_desired, dl_leg_desired, ddl_leg_desired, min_leg_length, max_leg_length);
end

== matlab function deadbeat_smm_with_lqr/Control/Behavior Control/Primary and Lateral Behavior/Flight/Calculate Time Until Touchdown ==
  data: z_dz input; t output; z_land parameter; g parameter
function t = EstimateTouchdown(z_dz, z_land, g)
  z_hat = z_dz(1); 
  dz_hat = z_dz(2);
  t = (-dz_hat-sqrt( max(dz_hat^2 - 4*g/2*(z_land-z_hat),0) ))/(-g);
end

== matlab function deadbeat_smm_with_lqr/Control/Behavior Control/Primary and Lateral Behavior/Flight/Convert COM Position to Joint Angles + Leg Length  ==
  data: hopping input; desired_leg_length output; X_star input; Y_star input; Z_star input; right_left input; com_pelvis_body input; desired_alpha output; desired_beta output; dcom_pelvis_body input; roll input; pitch input; sagittal_angle input; lateral_angle input; leg_length input; lateral_offset parameter; desired_initial_leg_roll_right parameter; desired_initial_leg_roll_left parameter; d_vertical_com parameter; desired_standing_z parameter; minimum_lateral_beta parameter; maximum_lateral_beta parameter
function [ desired_leg_length, desired_alpha, desired_beta ]  =  ...
          ConvertToJointAnglesAndLegLength(hopping, X_star, Y_star, Z_star, right_left,...
                           com_pelvis_body, dcom_pelvis_body, ...
                           roll, pitch, sagittal_angle, lateral_angle, leg_length,...
                           lateral_offset, desired_initial_leg_roll_right, desired_initial_leg_roll_left, d_vertical_com, desired_standing_z, ...
                           minimum_lateral_beta, maximum_lateral_beta) 

                                   
    q = [roll(1), pitch(1), sagittal_angle(1), lateral_angle(1), leg_length(1)];
    dq = [roll(2), pitch(2), sagittal_angle(2), lateral_angle(2), leg_length(2)];
    [desired_alpha, desired_beta, desired_leg_length]  =  ConvertComPositionToLegAnglesAndLegLength(X_star, Y_star, Z_star, right_left, com_pelvis_body, dcom_pelvis_body, q, dq, lateral_offset);   
                       
    if ~hopping
        desired_leg_length = [desired_standing_z-d_vertical_com; 0; 0];
        desired_alpha = [pi - pitch(1); -pitch(2); 0];
        desired_beta = [desired_initial_leg_roll_left; 0; 0];
        if right_left
            desired_beta = [desired_initial_leg_roll_right; 0; 0];
        end
    end
    desired_beta = saturate(desired_beta, minimum_lateral_beta, maximum_lateral_beta);
end

function [desired_saturated] = saturate(desired, minimum_lateral_beta, maximum_lateral_beta)
    desired_saturated = desired;
    if desired(1) < minimum_lateral_beta
        desired_saturated = [minimum_lateral_beta; 0; 0];
    elseif desired(1) > maximum_lateral_beta
        desired_saturated = [maximum_lateral_beta; 0; 0];    
    end
end
